simulink model "wtm2"  (R2020a)
settings: Solver=VariableStepAuto  StartTime=0.0  StopTime=10.0  RelTol=1e-3
(part 1 of 8)
settings Model: Creator=kishan  LastModifiedBy=kishan

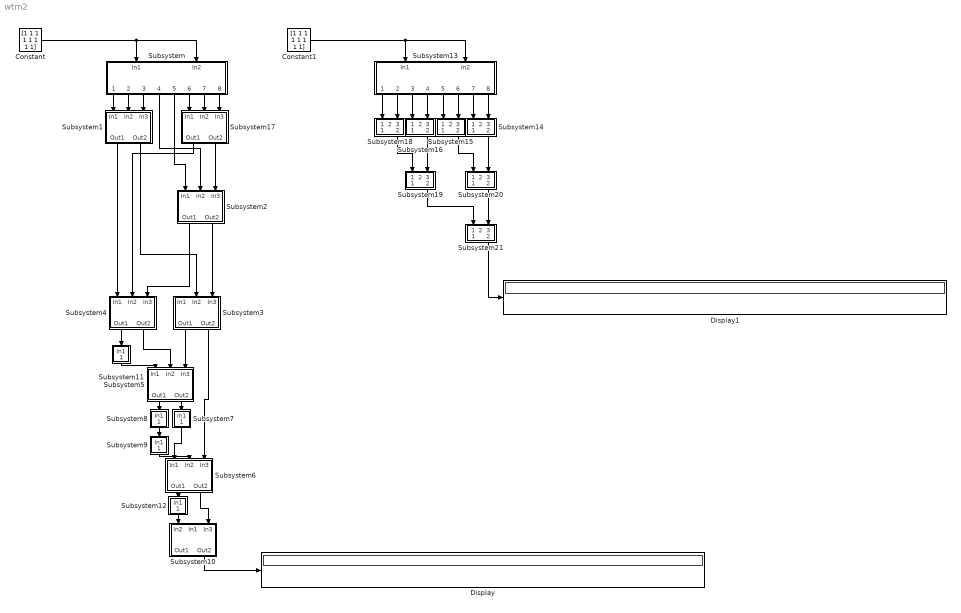
== system wtm2 ==
  Constant : Constant  Value=[1 1 1 1 1 1 1 1]  OutDataTypeStr=boolean
  Constant1 : Constant  Value=[1 1 1 1 1 1 1 1]  OutDataTypeStr=boolean
  Display : Display
  Display1 : Display
  Subsystem : Subsystem
  Subsystem1 : Subsystem
  Subsystem10 : Subsystem
  Subsystem11 : Subsystem
  Subsystem12 : Subsystem
  Subsystem13 : Subsystem
  Subsystem14 : Subsystem
  Subsystem15 : Subsystem
  Subsystem16 : Subsystem
  Subsystem17 : Subsystem
  Subsystem18 : Subsystem
  Subsystem19 : Subsystem
  Subsystem2 : Subsystem
  Subsystem20 : Subsystem
  Subsystem21 : Subsystem
  Subsystem3 : Subsystem
  Subsystem4 : Subsystem
  Subsystem5 : Subsystem
  Subsystem6 : Subsystem
  Subsystem7 : Subsystem
  Subsystem8 : Subsystem
  Subsystem9 : Subsystem
  wires:
  Subsystem/6(Out6) -> Subsystem17/1(In1)
  Subsystem/7(Out7) -> Subsystem17/2(In2)
  Subsystem/8(Out8) -> Subsystem17/3(In3)
  Constant/1 -> Subsystem/2(In2), Subsystem/1(In1)
  Subsystem10/2(Out2) -> Display/1
  Constant1/1 -> Subsystem13/2(In2), Subsystem13/1(In1)
  Subsystem13/8(Out8) -> Subsystem14/3(In3)
  Subsystem13/7(Out7) -> Subsystem14/1(In2)
  Subsystem13/6(Out6) -> Subsystem15/3(In3)
  Subsystem13/5(Out5) -> Subsystem15/1(In2)
  Subsystem13/4(Out4) -> Subsystem16/3(In3)
  Subsystem13/3(Out3) -> Subsystem16/1(In2)
  Subsystem13/2(Out2) -> Subsystem18/3(In3)
  Subsystem13/1(Out1) -> Subsystem18/1(In2)
  Subsystem16/2(Out2) -> Subsystem19/3(In3)
  Subsystem18/2(Out2) -> Subsystem19/1(In2)
  Subsystem14/2(Out2) -> Subsystem20/3(In3)
  Subsystem15/2(Out2) -> Subsystem20/1(In2)
  Subsystem20/2(Out2) -> Subsystem21/3(In3)
  Subsystem19/2(Out2) -> Subsystem21/1(In2)
  Subsystem21/2(Out2) -> Display1/1
  Subsystem/1(Out1) -> Subsystem1/1(In1)
  Subsystem/2(Out2) -> Subsystem1/2(In2)
  Subsystem/3(Out3) -> Subsystem1/3(In3)
  Subsystem17/2(Out2) -> Subsystem2/3(In3)
  Subsystem/5(Out5) -> Subsystem2/1(In1)
  Subsystem2/2(Out2) -> Subsystem3/3(In3)
  Subsystem1/1(Out1) -> Subsystem4/1(In1)
  Subsystem17/1(Out1) -> Subsystem4/2(In2)
  Subsystem2/1(Out1) -> Subsystem4/3(In3)
  Subsystem3/1(Out1) -> Subsystem5/3(In3)
  Subsystem4/2(Out2) -> Subsystem5/2(In2)
  Subsystem4/1(Out1) -> Subsystem11/1(In1)
  Subsystem11/1(Out2) -> Subsystem5/1(In1)
  Subsystem3/2(Out2) -> Subsystem6/3(In3)
  Subsystem5/2(Out2) -> Subsystem7/1(In1)
  Subsystem7/1(Out2) -> Subsystem6/1(In1)
  Subsystem5/1(Out1) -> Subsystem8/1(In1)
  Subsystem8/1(Out2) -> Subsystem9/1(In1)
  Subsystem9/1(Out2) -> Subsystem6/2(In2)
  Subsystem6/2(Out2) -> Subsystem10/3(In3)
  Subsystem6/1(Out1) -> Subsystem12/1(In1)
  Subsystem12/1(Out2) -> Subsystem10/1(In2)
  Subsystem/4(Out4) -> Subsystem2/2(In2)
  Subsystem1/2(Out2) -> Subsystem3/2(In2)

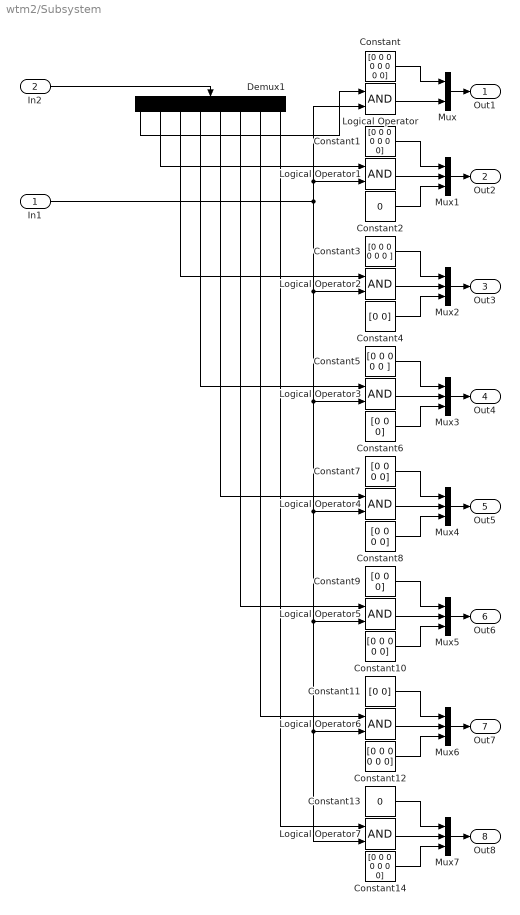
== system wtm2/Subsystem ==
  In1 : Inport
  In2 : Inport  Port=2
  Constant : Constant  Value=[0 0 0 0 0 0 0 0]  OutDataTypeStr=boolean
  Constant1 : Constant  Value=[0 0 0 0 0 0 0]  OutDataTypeStr=boolean
  Constant10 : Constant  Value=[0 0 0 0 0]  OutDataTypeStr=boolean
  Constant11 : Constant  Value=[0 0]  OutDataTypeStr=boolean
  Constant12 : Constant  Value=[0 0 0 0 0 0]  OutDataTypeStr=boolean
  Constant13 : Constant  Value=0  OutDataTypeStr=boolean
  Constant14 : Constant  Value=[0 0 0 0 0 0 0]  OutDataTypeStr=boolean
  Constant2 : Constant  Value=0  OutDataTypeStr=boolean
  Constant3 : Constant  Value=[0 0 0 0 0 0 ]  OutDataTypeStr=boolean
  Constant4 : Constant  Value=[0 0]  OutDataTypeStr=boolean
  Constant5 : Constant  Value=[0 0 0 0 0 ]  OutDataTypeStr=boolean
  Constant6 : Constant  Value=[0 0 0]  OutDataTypeStr=boolean
  Constant7 : Constant  Value=[0 0 0 0]  OutDataTypeStr=boolean
  Constant8 : Constant  Value=[0 0 0 0]  OutDataTypeStr=boolean
  Constant9 : Constant  Value=[0 0 0]  OutDataTypeStr=boolean
  Demux1 : Demux  Outputs=8
  Logical Operator{,1..7} (8 alike) : Logic  AllPortsSameDT=off  OutDataTypeStr=boolean
  Mux : Mux  Inputs=2
  Mux{1..7} (7 alike) : Mux  Inputs=3
  Out1 : Outport
  Out2 : Outport  Port=2
  Out3 : Outport  Port=3
  Out4 : Outport  Port=4
  Out5 : Outport  Port=5
  Out6 : Outport  Port=6
  Out7 : Outport  Port=7
  Out8 : Outport  Port=8
  wires:
  In2/1 -> Demux1/1
  In1/1 -> Logical Operator/2, Logical Operator1/2, Logical Operator2/2, Logical Operator3/2, Logical Operator4/2, Logical Operator5/2, Logical Operator7/2, Logical Operator6/2
  Constant7/1 -> Mux4/1
  Mux3/1 -> Out4/1
  Mux5/1 -> Out6/1
  Constant11/1 -> Mux6/1
  Constant2/1 -> Mux1/3
  Logical Operator3/1 -> Mux3/2
  Mux2/1 -> Out3/1
  Logical Operator2/1 -> Mux2/2
  Constant10/1 -> Mux5/3
  Constant/1 -> Mux/1
  Constant9/1 -> Mux5/1
  Constant4/1 -> Mux2/3
  Constant12/1 -> Mux6/3
  Logical Operator7/1 -> Mux7/2
  Constant8/1 -> Mux4/3
  Constant13/1 -> Mux7/1
  Constant14/1 -> Mux7/3
  Mux1/1 -> Out2/1
  Constant5/1 -> Mux3/1
  Mux6/1 -> Out7/1
  Constant1/1 -> Mux1/1
  Constant3/1 -> Mux2/1
  Mux/1 -> Out1/1
  Logical Operator6/1 -> Mux6/2
  Logical Operator/1 -> Mux/2
  Logical Operator4/1 -> Mux4/2
  Mux7/1 -> Out8/1
  Logical Operator1/1 -> Mux1/2
  Logical Operator5/1 -> Mux5/2
  Mux4/1 -> Out5/1
  Constant6/1 -> Mux3/3
  Demux1/8 -> Logical Operator7/1
  Demux1/7 -> Logical Operator6/1
  Demux1/6 -> Logical Operator5/1
  Demux1/5 -> Logical Operator4/1
  Demux1/4 -> Logical Operator3/1
  Demux1/3 -> Logical Operator2/1
  Demux1/2 -> Logical Operator1/1
  Demux1/1 -> Logical Operator/1

== system wtm2/Subsystem1 ==
  In1 : Inport
  In2 : Inport  Port=2
  In3 : Inport  Port=3
  Demux : Demux  Outputs=16
  Demux1 : Demux  Outputs=16
  Demux2 : Demux  Outputs=16
  Mux : Mux  Inputs=16
  Mux1 : Mux  Inputs=16
  Subsystem1 : Subsystem
  Subsystem10 : Subsystem
  Subsystem11 : Subsystem
  Subsystem12 : Subsystem
  Subsystem13 : Subsystem
  Subsystem14 : Subsystem
  Subsystem15 : Subsystem
  Subsystem16 : Subsystem
  Subsystem2 : Subsystem
  Subsystem3 : Subsystem
  Subsystem4 : Subsystem
  Subsystem5 : Subsystem
  Subsystem6 : Subsystem
  Subsystem7 : Subsystem
  Subsystem8 : Subsystem
  Subsystem9 : Subsystem
  Out1 : Outport
  Out2 : Outport  Port=2
  wires:
  Demux2/2 -> Subsystem2/3(In3)
  Demux/9 -> Subsystem9/1(In1)
  Subsystem7/1(Out1) -> Mux1/7
  Subsystem11/2(Out2) -> Mux/11
  Demux2/8 -> Subsystem8/3(In3)
  Subsystem2/2(Out2) -> Mux/2
  Subsystem1/2(Out2) -> Mux/1
  Demux/7 -> Subsystem7/1(In1)
  Demux2/11 -> Subsystem11/3(In3)
  Demux2/1 -> Subsystem1/3(In3)
  Demux1/10 -> Subsystem10/2(In2)
  Demux2/13 -> Subsystem13/3(In3)
  Subsystem4/2(Out2) -> Mux/4
  Demux1/16 -> Subsystem16/2(In2)
  Demux2/15 -> Subsystem15/3(In3)
  Demux2/3 -> Subsystem3/3(In3)
  Demux2/6 -> Subsystem6/3(In3)
  Mux1/1 -> Out2/1
  Demux/13 -> Subsystem13/1(In1)
  Subsystem14/1(Out1) -> Mux1/14
  Demux1/13 -> Subsystem13/2(In2)
  Subsystem12/1(Out1) -> Mux1/12
  Subsystem1/1(Out1) -> Mux1/1
  Demux1/2 -> Subsystem2/2(In2)
  Subsystem12/2(Out2) -> Mux/12
  Subsystem5/1(Out1) -> Mux1/5
  Demux2/12 -> Subsystem12/3(In3)
  Demux1/14 -> Subsystem14/2(In2)
  Subsystem13/1(Out1) -> Mux1/13
  Demux1/11 -> Subsystem11/2(In2)
  Subsystem7/2(Out2) -> Mux/7
  Demux2/5 -> Subsystem5/3(In3)
  Subsystem10/2(Out2) -> Mux/10
  Demux1/1 -> Subsystem1/2(In2)
  Demux2/10 -> Subsystem10/3(In3)
  Demux1/7 -> Subsystem7/2(In2)
  Subsystem16/1(Out1) -> Mux1/16
  Demux/3 -> Subsystem3/1(In1)
  Demux/14 -> Subsystem14/1(In1)
  Subsystem13/2(Out2) -> Mux/13
  Demux/6 -> Subsystem6/1(In1)
  Demux/11 -> Subsystem11/1(In1)
  Mux/1 -> Out1/1
  Subsystem3/2(Out2) -> Mux/3
  Subsystem2/1(Out1) -> Mux1/2
  Subsystem16/2(Out2) -> Mux/16
  Subsystem9/2(Out2) -> Mux/9
  Subsystem10/1(Out1) -> Mux1/10
  Subsystem6/2(Out2) -> Mux/6
  Demux/2 -> Subsystem2/1(In1)
  Demux1/12 -> Subsystem12/2(In2)
  Demux1/15 -> Subsystem15/2(In2)
  Demux2/14 -> Subsystem14/3(In3)
  Demux1/9 -> Subsystem9/2(In2)
  Subsystem4/1(Out1) -> Mux1/4
  Demux1/8 -> Subsystem8/2(In2)
  Demux/12 -> Subsystem12/1(In1)
  Subsystem3/1(Out1) -> Mux1/3
  In1/1 -> Demux2/1
  In2/1 -> Demux1/1
  Demux/8 -> Subsystem8/1(In1)
  Demux2/16 -> Subsystem16/3(In3)
  Demux1/6 -> Subsystem6/2(In2)
  Subsystem14/2(Out2) -> Mux/14
  Demux1/4 -> Subsystem4/2(In2)
  Demux/16 -> Subsystem16/1(In1)
  Subsystem9/1(Out1) -> Mux1/9
  Demux/4 -> Subsystem4/1(In1)
  Demux/15 -> Subsystem15/1(In1)
  Subsystem5/2(Out2) -> Mux/5
  Demux/1 -> Subsystem1/1(In1)
  Demux1/5 -> Subsystem5/2(In2)
  Subsystem15/1(Out1) -> Mux1/15
  Demux/10 -> Subsystem10/1(In1)
  Subsystem15/2(Out2) -> Mux/15
  Demux2/9 -> Subsystem9/3(In3)
  Subsystem6/1(Out1) -> Mux1/6
  Subsystem8/2(Out2) -> Mux/8
  Subsystem8/1(Out1) -> Mux1/8
  Demux2/7 -> Subsystem7/3(In3)
  In3/1 -> Demux/1
  Subsystem11/1(Out1) -> Mux1/11
  Demux1/3 -> Subsystem3/2(In2)
  Demux2/4 -> Subsystem4/3(In3)
  Demux/5 -> Subsystem5/1(In1)

== system wtm2/Subsystem10 ==
  In2 : Inport
  In1 : Inport  Port=2
  In3 : Inport  Port=3
  Demux : Demux  Outputs=16
  Demux1 : Demux  Outputs=16
  Mux : Mux  Inputs=16
  Subsystem4 : Subsystem
  Subsystem5 : Subsystem
  Subsystem6 : Subsystem
  Subsystem7 : Subsystem
  Out1 : Outport
  Out2 : Outport  Port=2
  wires:
  Demux/11 -> Subsystem5/3(In3)
  Subsystem4/4(Out4) -> Mux/15
  Demux1/4 -> Subsystem7/9(In9)
  Demux/14 -> Subsystem4/2(In2)
  Subsystem7/4(Out4) -> Mux/3
  Subsystem7/1(Out1) -> Out1/1
  Subsystem7/3(Out3) -> Mux/2
  Demux/3 -> Subsystem7/3(In3)
  Demux/15 -> Subsystem4/3(In3)
  Subsystem6/1(Out1) -> Subsystem7/5(In5)
  In3/1 -> Demux1/1
  Subsystem4/5(Out5) -> Mux/16
  Subsystem4/3(Out3) -> Mux/14
  Demux1/15 -> Subsystem4/8(In8)
  Subsystem5/4(Out4) -> Mux/11
  Subsystem5/1(Out1) -> Subsystem6/5(In5)
  Subsystem5/3(Out3) -> Mux/10
  Demux1/16 -> Subsystem4/9(In9)
  Demux/9 -> Subsystem5/1(In1)
  Subsystem7/5(Out5) -> Mux/4
  Demux1/3 -> Subsystem7/8(In8)
  Demux1/9 -> Subsystem5/6(In6)
  Subsystem6/5(Out5) -> Mux/8
  Demux/1 -> Subsystem7/1(In1)
  Demux1/13 -> Subsystem4/6(In6)
  Demux/5 -> Subsystem6/1(In1)
  Demux1/7 -> Subsystem6/8(In8)
  In2/1 -> Demux/1
  Demux1/12 -> Subsystem5/9(In9)
  Subsystem6/4(Out4) -> Mux/7
  Subsystem5/5(Out5) -> Mux/12
  Mux/1 -> Out2/1
  Subsystem6/3(Out3) -> Mux/6
  Demux1/8 -> Subsystem6/9(In9)
  Demux/12 -> Subsystem5/4(In4)
  Subsystem4/1(Out1) -> Subsystem5/5(In5)
  Demux/6 -> Subsystem6/2(In2)
  Subsystem6/2(Out2) -> Mux/5
  Demux1/1 -> Subsystem7/6(In6)
  Demux/8 -> Subsystem6/4(In4)
  Demux1/5 -> Subsystem6/6(In6)
  Demux/7 -> Subsystem6/3(In3)
  Demux/4 -> Subsystem7/4(In4)
  Demux/10 -> Subsystem5/2(In2)
  Subsystem5/2(Out2) -> Mux/9
  Demux/2 -> Subsystem7/2(In2)
  Demux1/6 -> Subsystem6/7(In7)
  Subsystem7/2(Out2) -> Mux/1
  Subsystem4/2(Out2) -> Mux/13
  Demux/13 -> Subsystem4/1(In1)
  Demux1/11 -> Subsystem5/8(In8)
  Demux1/2 -> Subsystem7/7(In7)
  Demux1/14 -> Subsystem4/7(In7)
  Demux/16 -> Subsystem4/4(In4)
  Demux1/10 -> Subsystem5/7(In7)
  In1/1 -> Subsystem4/5(In5)

== system wtm2/Subsystem11 ==
  In1 : Inport
  Constant : Constant  Value=0  OutDataTypeStr=boolean
  Demux : Demux  Outputs=16
  Display : Display
  Mux : Mux  Inputs=16
  Out2 : Outport
  wires:
  Demux/5 -> Mux/6
  Demux/6 -> Mux/7
  Demux/4 -> Mux/5
  Demux/10 -> Mux/11
  In1/1 -> Demux/1
  Constant/1 -> Mux/1
  Demux/15 -> Mux/16
  Mux/1 -> Out2/1
  Demux/1 -> Mux/2
  Demux/9 -> Mux/10
  Demux/2 -> Mux/3
  Demux/11 -> Mux/12
  Demux/12 -> Mux/13
  Demux/14 -> Mux/15
  Demux/13 -> Mux/14
  Demux/3 -> Mux/4
  Demux/8 -> Mux/9
  Demux/7 -> Mux/8
  Demux/16 -> Display/1

== system wtm2/Subsystem12 ==
  In1 : Inport
  Constant : Constant  Value=0  OutDataTypeStr=boolean
  Demux : Demux  Outputs=16
  Display : Display
  Mux : Mux  Inputs=16
  Out2 : Outport
  wires:
  Demux/5 -> Mux/6
  Demux/6 -> Mux/7
  Demux/4 -> Mux/5
  Demux/10 -> Mux/11
  In1/1 -> Demux/1
  Constant/1 -> Mux/1
  Demux/15 -> Mux/16
  Mux/1 -> Out2/1
  Demux/1 -> Mux/2
  Demux/9 -> Mux/10
  Demux/2 -> Mux/3
  Demux/11 -> Mux/12
  Demux/12 -> Mux/13
  Demux/14 -> Mux/15
  Demux/13 -> Mux/14
  Demux/3 -> Mux/4
  Demux/8 -> Mux/9
  Demux/7 -> Mux/8
  Demux/16 -> Display/1

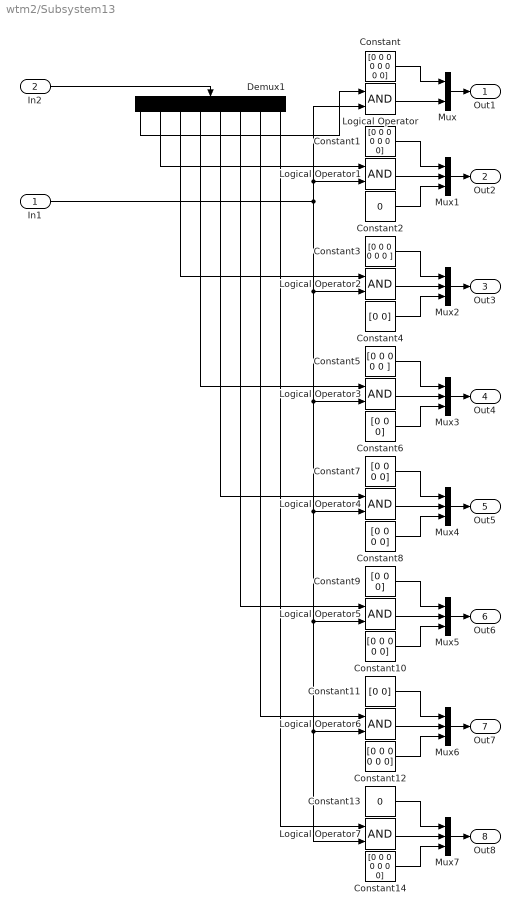
== system wtm2/Subsystem13 ==
  In1 : Inport
  In2 : Inport  Port=2
  Constant : Constant  Value=[0 0 0 0 0 0 0 0]  OutDataTypeStr=boolean
  Constant1 : Constant  Value=[0 0 0 0 0 0 0]  OutDataTypeStr=boolean
  Constant10 : Constant  Value=[0 0 0 0 0]  OutDataTypeStr=boolean
  Constant11 : Constant  Value=[0 0]  OutDataTypeStr=boolean
  Constant12 : Constant  Value=[0 0 0 0 0 0]  OutDataTypeStr=boolean
  Constant13 : Constant  Value=0  OutDataTypeStr=boolean
  Constant14 : Constant  Value=[0 0 0 0 0 0 0]  OutDataTypeStr=boolean
  Constant2 : Constant  Value=0  OutDataTypeStr=boolean
  Constant3 : Constant  Value=[0 0 0 0 0 0 ]  OutDataTypeStr=boolean
  Constant4 : Constant  Value=[0 0]  OutDataTypeStr=boolean
  Constant5 : Constant  Value=[0 0 0 0 0 ]  OutDataTypeStr=boolean
  Constant6 : Constant  Value=[0 0 0]  OutDataTypeStr=boolean
  Constant7 : Constant  Value=[0 0 0 0]  OutDataTypeStr=boolean
  Constant8 : Constant  Value=[0 0 0 0]  OutDataTypeStr=boolean
  Constant9 : Constant  Value=[0 0 0]  OutDataTypeStr=boolean
  Demux1 : Demux  Outputs=8
  Logical Operator{,1..7} (8 alike) : Logic  AllPortsSameDT=off  OutDataTypeStr=boolean
  Mux : Mux  Inputs=2
  Mux{1..7} (7 alike) : Mux  Inputs=3
  Out1 : Outport
  Out2 : Outport  Port=2
  Out3 : Outport  Port=3
  Out4 : Outport  Port=4
  Out5 : Outport  Port=5
  Out6 : Outport  Port=6
  Out7 : Outport  Port=7
  Out8 : Outport  Port=8
  wires:
  In2/1 -> Demux1/1
  In1/1 -> Logical Operator/2, Logical Operator1/2, Logical Operator2/2, Logical Operator3/2, Logical Operator4/2, Logical Operator5/2, Logical Operator7/2, Logical Operator6/2
  Constant7/1 -> Mux4/1
  Mux3/1 -> Out4/1
  Mux5/1 -> Out6/1
  Constant11/1 -> Mux6/1
  Constant2/1 -> Mux1/3
  Logical Operator3/1 -> Mux3/2
  Mux2/1 -> Out3/1
  Logical Operator2/1 -> Mux2/2
  Constant10/1 -> Mux5/3
  Constant/1 -> Mux/1
  Constant9/1 -> Mux5/1
  Constant4/1 -> Mux2/3
  Constant12/1 -> Mux6/3
  Logical Operator7/1 -> Mux7/2
  Constant8/1 -> Mux4/3
  Constant13/1 -> Mux7/1
  Constant14/1 -> Mux7/3
  Mux1/1 -> Out2/1
  Constant5/1 -> Mux3/1
  Mux6/1 -> Out7/1
  Constant1/1 -> Mux1/1
  Constant3/1 -> Mux2/1
  Mux/1 -> Out1/1
  Logical Operator6/1 -> Mux6/2
  Logical Operator/1 -> Mux/2
  Logical Operator4/1 -> Mux4/2
  Mux7/1 -> Out8/1
  Logical Operator1/1 -> Mux1/2
  Logical Operator5/1 -> Mux5/2
  Mux4/1 -> Out5/1
  Constant6/1 -> Mux3/3
  Demux1/8 -> Logical Operator7/1
  Demux1/7 -> Logical Operator6/1
  Demux1/6 -> Logical Operator5/1
  Demux1/5 -> Logical Operator4/1
  Demux1/4 -> Logical Operator3/1
  Demux1/3 -> Logical Operator2/1
  Demux1/2 -> Logical Operator1/1
  Demux1/1 -> Logical Operator/1

== system wtm2/Subsystem14 ==
  In2 : Inport
  In1 : Inport  Port=2
  In3 : Inport  Port=3
  Demux : Demux  Outputs=16
  Demux1 : Demux  Outputs=16
  Mux : Mux  Inputs=16
  Subsystem4 : Subsystem
  Subsystem5 : Subsystem
  Subsystem6 : Subsystem
  Subsystem7 : Subsystem
  Out1 : Outport
  Out2 : Outport  Port=2
  wires:
  Demux/11 -> Subsystem5/3(In3)
  Subsystem4/4(Out4) -> Mux/15
  Demux1/4 -> Subsystem7/9(In9)
  Demux/14 -> Subsystem4/2(In2)
  Subsystem7/4(Out4) -> Mux/3
  Subsystem7/1(Out1) -> Out1/1
  Subsystem7/3(Out3) -> Mux/2
  Demux/3 -> Subsystem7/3(In3)
  Demux/15 -> Subsystem4/3(In3)
  Subsystem6/1(Out1) -> Subsystem7/5(In5)
  In3/1 -> Demux1/1
  Subsystem4/5(Out5) -> Mux/16
  Subsystem4/3(Out3) -> Mux/14
  Demux1/15 -> Subsystem4/8(In8)
  Subsystem5/4(Out4) -> Mux/11
  Subsystem5/1(Out1) -> Subsystem6/5(In5)
  Subsystem5/3(Out3) -> Mux/10
  Demux1/16 -> Subsystem4/9(In9)
  Demux/9 -> Subsystem5/1(In1)
  Subsystem7/5(Out5) -> Mux/4
  Demux1/3 -> Subsystem7/8(In8)
  Demux1/9 -> Subsystem5/6(In6)
  Subsystem6/5(Out5) -> Mux/8
  Demux/1 -> Subsystem7/1(In1)
  Demux1/13 -> Subsystem4/6(In6)
  Demux/5 -> Subsystem6/1(In1)
  Demux1/7 -> Subsystem6/8(In8)
  In2/1 -> Demux/1
  Demux1/12 -> Subsystem5/9(In9)
  Subsystem6/4(Out4) -> Mux/7
  Subsystem5/5(Out5) -> Mux/12
  Mux/1 -> Out2/1
  Subsystem6/3(Out3) -> Mux/6
  Demux1/8 -> Subsystem6/9(In9)
  Demux/12 -> Subsystem5/4(In4)
  Subsystem4/1(Out1) -> Subsystem5/5(In5)
  Demux/6 -> Subsystem6/2(In2)
  Subsystem6/2(Out2) -> Mux/5
  Demux1/1 -> Subsystem7/6(In6)
  Demux/8 -> Subsystem6/4(In4)
  Demux1/5 -> Subsystem6/6(In6)
  Demux/7 -> Subsystem6/3(In3)
  Demux/4 -> Subsystem7/4(In4)
  Demux/10 -> Subsystem5/2(In2)
  Subsystem5/2(Out2) -> Mux/9
  Demux/2 -> Subsystem7/2(In2)
  Demux1/6 -> Subsystem6/7(In7)
  Subsystem7/2(Out2) -> Mux/1
  Subsystem4/2(Out2) -> Mux/13
  Demux/13 -> Subsystem4/1(In1)
  Demux1/11 -> Subsystem5/8(In8)
  Demux1/2 -> Subsystem7/7(In7)
  Demux1/14 -> Subsystem4/7(In7)
  Demux/16 -> Subsystem4/4(In4)
  Demux1/10 -> Subsystem5/7(In7)
  In1/1 -> Subsystem4/5(In5)

== system wtm2/Subsystem15 ==
  In2 : Inport
  In1 : Inport  Port=2
  In3 : Inport  Port=3
  Demux : Demux  Outputs=16
  Demux1 : Demux  Outputs=16
  Mux : Mux  Inputs=16
  Subsystem4 : Subsystem
  Subsystem5 : Subsystem
  Subsystem6 : Subsystem
  Subsystem7 : Subsystem
  Out1 : Outport
  Out2 : Outport  Port=2
  wires:
  Demux/11 -> Subsystem5/3(In3)
  Subsystem4/4(Out4) -> Mux/15
  Demux1/4 -> Subsystem7/9(In9)
  Demux/14 -> Subsystem4/2(In2)
  Subsystem7/4(Out4) -> Mux/3
  Subsystem7/1(Out1) -> Out1/1
  Subsystem7/3(Out3) -> Mux/2
  Demux/3 -> Subsystem7/3(In3)
  Demux/15 -> Subsystem4/3(In3)
  Subsystem6/1(Out1) -> Subsystem7/5(In5)
  In3/1 -> Demux1/1
  Subsystem4/5(Out5) -> Mux/16
  Subsystem4/3(Out3) -> Mux/14
  Demux1/15 -> Subsystem4/8(In8)
  Subsystem5/4(Out4) -> Mux/11
  Subsystem5/1(Out1) -> Subsystem6/5(In5)
  Subsystem5/3(Out3) -> Mux/10
  Demux1/16 -> Subsystem4/9(In9)
  Demux/9 -> Subsystem5/1(In1)
  Subsystem7/5(Out5) -> Mux/4
  Demux1/3 -> Subsystem7/8(In8)
  Demux1/9 -> Subsystem5/6(In6)
  Subsystem6/5(Out5) -> Mux/8
  Demux/1 -> Subsystem7/1(In1)
  Demux1/13 -> Subsystem4/6(In6)
  Demux/5 -> Subsystem6/1(In1)
  Demux1/7 -> Subsystem6/8(In8)
  In2/1 -> Demux/1
  Demux1/12 -> Subsystem5/9(In9)
  Subsystem6/4(Out4) -> Mux/7
  Subsystem5/5(Out5) -> Mux/12
  Mux/1 -> Out2/1
  Subsystem6/3(Out3) -> Mux/6
  Demux1/8 -> Subsystem6/9(In9)
  Demux/12 -> Subsystem5/4(In4)
  Subsystem4/1(Out1) -> Subsystem5/5(In5)
  Demux/6 -> Subsystem6/2(In2)
  Subsystem6/2(Out2) -> Mux/5
  Demux1/1 -> Subsystem7/6(In6)
  Demux/8 -> Subsystem6/4(In4)
  Demux1/5 -> Subsystem6/6(In6)
  Demux/7 -> Subsystem6/3(In3)
  Demux/4 -> Subsystem7/4(In4)
  Demux/10 -> Subsystem5/2(In2)
  Subsystem5/2(Out2) -> Mux/9
  Demux/2 -> Subsystem7/2(In2)
  Demux1/6 -> Subsystem6/7(In7)
  Subsystem7/2(Out2) -> Mux/1
  Subsystem4/2(Out2) -> Mux/13
  Demux/13 -> Subsystem4/1(In1)
  Demux1/11 -> Subsystem5/8(In8)
  Demux1/2 -> Subsystem7/7(In7)
  Demux1/14 -> Subsystem4/7(In7)
  Demux/16 -> Subsystem4/4(In4)
  Demux1/10 -> Subsystem5/7(In7)
  In1/1 -> Subsystem4/5(In5)

== system wtm2/Subsystem16 ==
  In2 : Inport
  In1 : Inport  Port=2
  In3 : Inport  Port=3
  Demux : Demux  Outputs=16
  Demux1 : Demux  Outputs=16
  Mux : Mux  Inputs=16
  Subsystem4 : Subsystem
  Subsystem5 : Subsystem
  Subsystem6 : Subsystem
  Subsystem7 : Subsystem
  Out1 : Outport
  Out2 : Outport  Port=2
  wires:
  Demux/11 -> Subsystem5/3(In3)
  Subsystem4/4(Out4) -> Mux/15
  Demux1/4 -> Subsystem7/9(In9)
  Demux/14 -> Subsystem4/2(In2)
  Subsystem7/4(Out4) -> Mux/3
  Subsystem7/1(Out1) -> Out1/1
  Subsystem7/3(Out3) -> Mux/2
  Demux/3 -> Subsystem7/3(In3)
  Demux/15 -> Subsystem4/3(In3)
  Subsystem6/1(Out1) -> Subsystem7/5(In5)
  In3/1 -> Demux1/1
  Subsystem4/5(Out5) -> Mux/16
  Subsystem4/3(Out3) -> Mux/14
  Demux1/15 -> Subsystem4/8(In8)
  Subsystem5/4(Out4) -> Mux/11
  Subsystem5/1(Out1) -> Subsystem6/5(In5)
  Subsystem5/3(Out3) -> Mux/10
  Demux1/16 -> Subsystem4/9(In9)
  Demux/9 -> Subsystem5/1(In1)
  Subsystem7/5(Out5) -> Mux/4
  Demux1/3 -> Subsystem7/8(In8)
  Demux1/9 -> Subsystem5/6(In6)
  Subsystem6/5(Out5) -> Mux/8
  Demux/1 -> Subsystem7/1(In1)
  Demux1/13 -> Subsystem4/6(In6)
  Demux/5 -> Subsystem6/1(In1)
  Demux1/7 -> Subsystem6/8(In8)
  In2/1 -> Demux/1
  Demux1/12 -> Subsystem5/9(In9)
  Subsystem6/4(Out4) -> Mux/7
  Subsystem5/5(Out5) -> Mux/12
  Mux/1 -> Out2/1
  Subsystem6/3(Out3) -> Mux/6
  Demux1/8 -> Subsystem6/9(In9)
  Demux/12 -> Subsystem5/4(In4)
  Subsystem4/1(Out1) -> Subsystem5/5(In5)
  Demux/6 -> Subsystem6/2(In2)
  Subsystem6/2(Out2) -> Mux/5
  Demux1/1 -> Subsystem7/6(In6)
  Demux/8 -> Subsystem6/4(In4)
  Demux1/5 -> Subsystem6/6(In6)
  Demux/7 -> Subsystem6/3(In3)
  Demux/4 -> Subsystem7/4(In4)
  Demux/10 -> Subsystem5/2(In2)
  Subsystem5/2(Out2) -> Mux/9
  Demux/2 -> Subsystem7/2(In2)
  Demux1/6 -> Subsystem6/7(In7)
  Subsystem7/2(Out2) -> Mux/1
  Subsystem4/2(Out2) -> Mux/13
  Demux/13 -> Subsystem4/1(In1)
  Demux1/11 -> Subsystem5/8(In8)
  Demux1/2 -> Subsystem7/7(In7)
  Demux1/14 -> Subsystem4/7(In7)
  Demux/16 -> Subsystem4/4(In4)
  Demux1/10 -> Subsystem5/7(In7)
  In1/1 -> Subsystem4/5(In5)

== system wtm2/Subsystem17 ==
  In1 : Inport
  In2 : Inport  Port=2
  In3 : Inport  Port=3
  Demux : Demux  Outputs=16
  Demux1 : Demux  Outputs=16
  Demux2 : Demux  Outputs=16
  Mux : Mux  Inputs=16
  Mux1 : Mux  Inputs=16
  Subsystem1 : Subsystem
  Subsystem10 : Subsystem
  Subsystem11 : Subsystem
  Subsystem12 : Subsystem
  Subsystem13 : Subsystem
  Subsystem14 : Subsystem
  Subsystem15 : Subsystem
  Subsystem16 : Subsystem
  Subsystem2 : Subsystem
  Subsystem3 : Subsystem
  Subsystem4 : Subsystem
  Subsystem5 : Subsystem
  Subsystem6 : Subsystem
  Subsystem7 : Subsystem
  Subsystem8 : Subsystem
  Subsystem9 : Subsystem
  Out1 : Outport
  Out2 : Outport  Port=2
  wires:
  Demux2/2 -> Subsystem2/3(In3)
  Demux/9 -> Subsystem9/1(In1)
  Subsystem7/1(Out1) -> Mux1/7
  Subsystem11/2(Out2) -> Mux/11
  Demux2/8 -> Subsystem8/3(In3)
  Subsystem2/2(Out2) -> Mux/2
  Subsystem1/2(Out2) -> Mux/1
  Demux/7 -> Subsystem7/1(In1)
  Demux2/11 -> Subsystem11/3(In3)
  Demux2/1 -> Subsystem1/3(In3)
  Demux1/10 -> Subsystem10/2(In2)
  Demux2/13 -> Subsystem13/3(In3)
  Subsystem4/2(Out2) -> Mux/4
  Demux1/16 -> Subsystem16/2(In2)
  Demux2/15 -> Subsystem15/3(In3)
  Demux2/3 -> Subsystem3/3(In3)
  Demux2/6 -> Subsystem6/3(In3)
  Mux1/1 -> Out2/1
  Demux/13 -> Subsystem13/1(In1)
  Subsystem14/1(Out1) -> Mux1/14
  Demux1/13 -> Subsystem13/2(In2)
  Subsystem12/1(Out1) -> Mux1/12
  Subsystem1/1(Out1) -> Mux1/1
  Demux1/2 -> Subsystem2/2(In2)
  Subsystem12/2(Out2) -> Mux/12
  Subsystem5/1(Out1) -> Mux1/5
  Demux2/12 -> Subsystem12/3(In3)
  Demux1/14 -> Subsystem14/2(In2)
  Subsystem13/1(Out1) -> Mux1/13
  Demux1/11 -> Subsystem11/2(In2)
  Subsystem7/2(Out2) -> Mux/7
  Demux2/5 -> Subsystem5/3(In3)
  Subsystem10/2(Out2) -> Mux/10
  Demux1/1 -> Subsystem1/2(In2)
  Demux2/10 -> Subsystem10/3(In3)
  Demux1/7 -> Subsystem7/2(In2)
  Subsystem16/1(Out1) -> Mux1/16
  Demux/3 -> Subsystem3/1(In1)
  Demux/14 -> Subsystem14/1(In1)
  Subsystem13/2(Out2) -> Mux/13
  Demux/6 -> Subsystem6/1(In1)
  Demux/11 -> Subsystem11/1(In1)
  Mux/1 -> Out1/1
  Subsystem3/2(Out2) -> Mux/3
  Subsystem2/1(Out1) -> Mux1/2
  Subsystem16/2(Out2) -> Mux/16
  Subsystem9/2(Out2) -> Mux/9
  Subsystem10/1(Out1) -> Mux1/10
  Subsystem6/2(Out2) -> Mux/6
  Demux/2 -> Subsystem2/1(In1)
  Demux1/12 -> Subsystem12/2(In2)
  Demux1/15 -> Subsystem15/2(In2)
  Demux2/14 -> Subsystem14/3(In3)
  Demux1/9 -> Subsystem9/2(In2)
  Subsystem4/1(Out1) -> Mux1/4
  Demux1/8 -> Subsystem8/2(In2)
  Demux/12 -> Subsystem12/1(In1)
  Subsystem3/1(Out1) -> Mux1/3
  In1/1 -> Demux2/1
  In2/1 -> Demux1/1
  Demux/8 -> Subsystem8/1(In1)
  Demux2/16 -> Subsystem16/3(In3)
  Demux1/6 -> Subsystem6/2(In2)
  Subsystem14/2(Out2) -> Mux/14
  Demux1/4 -> Subsystem4/2(In2)
  Demux/16 -> Subsystem16/1(In1)
  Subsystem9/1(Out1) -> Mux1/9
  Demux/4 -> Subsystem4/1(In1)
  Demux/15 -> Subsystem15/1(In1)
  Subsystem5/2(Out2) -> Mux/5
  Demux/1 -> Subsystem1/1(In1)
  Demux1/5 -> Subsystem5/2(In2)
  Subsystem15/1(Out1) -> Mux1/15
  Demux/10 -> Subsystem10/1(In1)
  Subsystem15/2(Out2) -> Mux/15
  Demux2/9 -> Subsystem9/3(In3)
  Subsystem6/1(Out1) -> Mux1/6
  Subsystem8/2(Out2) -> Mux/8
  Subsystem8/1(Out1) -> Mux1/8
  Demux2/7 -> Subsystem7/3(In3)
  In3/1 -> Demux/1
  Subsystem11/1(Out1) -> Mux1/11
  Demux1/3 -> Subsystem3/2(In2)
  Demux2/4 -> Subsystem4/3(In3)
  Demux/5 -> Subsystem5/1(In1)

== system wtm2/Subsystem18 ==
  In2 : Inport
  In1 : Inport  Port=2
  In3 : Inport  Port=3
  Demux : Demux  Outputs=16
  Demux1 : Demux  Outputs=16
  Mux : Mux  Inputs=16
  Subsystem4 : Subsystem
  Subsystem5 : Subsystem
  Subsystem6 : Subsystem
  Subsystem7 : Subsystem
  Out1 : Outport
  Out2 : Outport  Port=2
  wires:
  Demux/11 -> Subsystem5/3(In3)
  Subsystem4/4(Out4) -> Mux/15
  Demux1/4 -> Subsystem7/9(In9)
  Demux/14 -> Subsystem4/2(In2)
  Subsystem7/4(Out4) -> Mux/3
  Subsystem7/1(Out1) -> Out1/1
  Subsystem7/3(Out3) -> Mux/2
  Demux/3 -> Subsystem7/3(In3)
  Demux/15 -> Subsystem4/3(In3)
  Subsystem6/1(Out1) -> Subsystem7/5(In5)
  In3/1 -> Demux1/1
  Subsystem4/5(Out5) -> Mux/16
  Subsystem4/3(Out3) -> Mux/14
  Demux1/15 -> Subsystem4/8(In8)
  Subsystem5/4(Out4) -> Mux/11
  Subsystem5/1(Out1) -> Subsystem6/5(In5)
  Subsystem5/3(Out3) -> Mux/10
  Demux1/16 -> Subsystem4/9(In9)
  Demux/9 -> Subsystem5/1(In1)
  Subsystem7/5(Out5) -> Mux/4
  Demux1/3 -> Subsystem7/8(In8)
  Demux1/9 -> Subsystem5/6(In6)
  Subsystem6/5(Out5) -> Mux/8
  Demux/1 -> Subsystem7/1(In1)
  Demux1/13 -> Subsystem4/6(In6)
  Demux/5 -> Subsystem6/1(In1)
  Demux1/7 -> Subsystem6/8(In8)
  In2/1 -> Demux/1
  Demux1/12 -> Subsystem5/9(In9)
  Subsystem6/4(Out4) -> Mux/7
  Subsystem5/5(Out5) -> Mux/12
  Mux/1 -> Out2/1
  Subsystem6/3(Out3) -> Mux/6
  Demux1/8 -> Subsystem6/9(In9)
  Demux/12 -> Subsystem5/4(In4)
  Subsystem4/1(Out1) -> Subsystem5/5(In5)
  Demux/6 -> Subsystem6/2(In2)
  Subsystem6/2(Out2) -> Mux/5
  Demux1/1 -> Subsystem7/6(In6)
  Demux/8 -> Subsystem6/4(In4)
  Demux1/5 -> Subsystem6/6(In6)
  Demux/7 -> Subsystem6/3(In3)
  Demux/4 -> Subsystem7/4(In4)
  Demux/10 -> Subsystem5/2(In2)
  Subsystem5/2(Out2) -> Mux/9
  Demux/2 -> Subsystem7/2(In2)
  Demux1/6 -> Subsystem6/7(In7)
  Subsystem7/2(Out2) -> Mux/1
  Subsystem4/2(Out2) -> Mux/13
  Demux/13 -> Subsystem4/1(In1)
  Demux1/11 -> Subsystem5/8(In8)
  Demux1/2 -> Subsystem7/7(In7)
  Demux1/14 -> Subsystem4/7(In7)
  Demux/16 -> Subsystem4/4(In4)
  Demux1/10 -> Subsystem5/7(In7)
  In1/1 -> Subsystem4/5(In5)

== system wtm2/Subsystem19 ==
  In2 : Inport
  In1 : Inport  Port=2
  In3 : Inport  Port=3
  Demux : Demux  Outputs=16
  Demux1 : Demux  Outputs=16
  Mux : Mux  Inputs=16
  Subsystem4 : Subsystem
  Subsystem5 : Subsystem
  Subsystem6 : Subsystem
  Subsystem7 : Subsystem
  Out1 : Outport
  Out2 : Outport  Port=2
  wires:
  Demux/11 -> Subsystem5/3(In3)
  Subsystem4/4(Out4) -> Mux/15
  Demux1/4 -> Subsystem7/9(In9)
  Demux/14 -> Subsystem4/2(In2)
  Subsystem7/4(Out4) -> Mux/3
  Subsystem7/1(Out1) -> Out1/1
  Subsystem7/3(Out3) -> Mux/2
  Demux/3 -> Subsystem7/3(In3)
  Demux/15 -> Subsystem4/3(In3)
  Subsystem6/1(Out1) -> Subsystem7/5(In5)
  In3/1 -> Demux1/1
  Subsystem4/5(Out5) -> Mux/16
  Subsystem4/3(Out3) -> Mux/14
  Demux1/15 -> Subsystem4/8(In8)
  Subsystem5/4(Out4) -> Mux/11
  Subsystem5/1(Out1) -> Subsystem6/5(In5)
  Subsystem5/3(Out3) -> Mux/10
  Demux1/16 -> Subsystem4/9(In9)
  Demux/9 -> Subsystem5/1(In1)
  Subsystem7/5(Out5) -> Mux/4
  Demux1/3 -> Subsystem7/8(In8)
  Demux1/9 -> Subsystem5/6(In6)
  Subsystem6/5(Out5) -> Mux/8
  Demux/1 -> Subsystem7/1(In1)
  Demux1/13 -> Subsystem4/6(In6)
  Demux/5 -> Subsystem6/1(In1)
  Demux1/7 -> Subsystem6/8(In8)
  In2/1 -> Demux/1
  Demux1/12 -> Subsystem5/9(In9)
  Subsystem6/4(Out4) -> Mux/7
  Subsystem5/5(Out5) -> Mux/12
  Mux/1 -> Out2/1
  Subsystem6/3(Out3) -> Mux/6
  Demux1/8 -> Subsystem6/9(In9)
  Demux/12 -> Subsystem5/4(In4)
  Subsystem4/1(Out1) -> Subsystem5/5(In5)
  Demux/6 -> Subsystem6/2(In2)
  Subsystem6/2(Out2) -> Mux/5
  Demux1/1 -> Subsystem7/6(In6)
  Demux/8 -> Subsystem6/4(In4)
  Demux1/5 -> Subsystem6/6(In6)
  Demux/7 -> Subsystem6/3(In3)
  Demux/4 -> Subsystem7/4(In4)
  Demux/10 -> Subsystem5/2(In2)
  Subsystem5/2(Out2) -> Mux/9
  Demux/2 -> Subsystem7/2(In2)
  Demux1/6 -> Subsystem6/7(In7)
  Subsystem7/2(Out2) -> Mux/1
  Subsystem4/2(Out2) -> Mux/13
  Demux/13 -> Subsystem4/1(In1)
  Demux1/11 -> Subsystem5/8(In8)
  Demux1/2 -> Subsystem7/7(In7)
  Demux1/14 -> Subsystem4/7(In7)
  Demux/16 -> Subsystem4/4(In4)
  Demux1/10 -> Subsystem5/7(In7)
  In1/1 -> Subsystem4/5(In5)

== system wtm2/Subsystem2 ==
  In1 : Inport
  In2 : Inport  Port=2
  In3 : Inport  Port=3
  Demux : Demux  Outputs=16
  Demux1 : Demux  Outputs=16
  Demux2 : Demux  Outputs=16
  Mux : Mux  Inputs=16
  Mux1 : Mux  Inputs=16
  Subsystem1 : Subsystem
  Subsystem10 : Subsystem
  Subsystem11 : Subsystem
  Subsystem12 : Subsystem
  Subsystem13 : Subsystem
  Subsystem14 : Subsystem
  Subsystem15 : Subsystem
  Subsystem16 : Subsystem
  Subsystem2 : Subsystem
  Subsystem3 : Subsystem
  Subsystem4 : Subsystem
  Subsystem5 : Subsystem
  Subsystem6 : Subsystem
  Subsystem7 : Subsystem
  Subsystem8 : Subsystem
  Subsystem9 : Subsystem
  Out1 : Outport
  Out2 : Outport  Port=2
  wires:
  Demux2/2 -> Subsystem2/3(In3)
  Demux/9 -> Subsystem9/1(In1)
  Subsystem7/1(Out1) -> Mux1/7
  Subsystem11/2(Out2) -> Mux/11
  Demux2/8 -> Subsystem8/3(In3)
  Subsystem2/2(Out2) -> Mux/2
  Subsystem1/2(Out2) -> Mux/1
  Demux/7 -> Subsystem7/1(In1)
  Demux2/11 -> Subsystem11/3(In3)
  Demux2/1 -> Subsystem1/3(In3)
  Demux1/10 -> Subsystem10/2(In2)
  Demux2/13 -> Subsystem13/3(In3)
  Subsystem4/2(Out2) -> Mux/4
  Demux1/16 -> Subsystem16/2(In2)
  Demux2/15 -> Subsystem15/3(In3)
  Demux2/3 -> Subsystem3/3(In3)
  Demux2/6 -> Subsystem6/3(In3)
  Mux1/1 -> Out2/1
  Demux/13 -> Subsystem13/1(In1)
  Subsystem14/1(Out1) -> Mux1/14
  Demux1/13 -> Subsystem13/2(In2)
  Subsystem12/1(Out1) -> Mux1/12
  Subsystem1/1(Out1) -> Mux1/1
  Demux1/2 -> Subsystem2/2(In2)
  Subsystem12/2(Out2) -> Mux/12
  Subsystem5/1(Out1) -> Mux1/5
  Demux2/12 -> Subsystem12/3(In3)
  Demux1/14 -> Subsystem14/2(In2)
  Subsystem13/1(Out1) -> Mux1/13
  Demux1/11 -> Subsystem11/2(In2)
  Subsystem7/2(Out2) -> Mux/7
  Demux2/5 -> Subsystem5/3(In3)
  Subsystem10/2(Out2) -> Mux/10
  Demux1/1 -> Subsystem1/2(In2)
  Demux2/10 -> Subsystem10/3(In3)
  Demux1/7 -> Subsystem7/2(In2)
  Subsystem16/1(Out1) -> Mux1/16
  Demux/3 -> Subsystem3/1(In1)
  Demux/14 -> Subsystem14/1(In1)
  Subsystem13/2(Out2) -> Mux/13
  Demux/6 -> Subsystem6/1(In1)
  Demux/11 -> Subsystem11/1(In1)
  Mux/1 -> Out1/1
  Subsystem3/2(Out2) -> Mux/3
  Subsystem2/1(Out1) -> Mux1/2
  Subsystem16/2(Out2) -> Mux/16
  Subsystem9/2(Out2) -> Mux/9
  Subsystem10/1(Out1) -> Mux1/10
  Subsystem6/2(Out2) -> Mux/6
  Demux/2 -> Subsystem2/1(In1)
  Demux1/12 -> Subsystem12/2(In2)
  Demux1/15 -> Subsystem15/2(In2)
  Demux2/14 -> Subsystem14/3(In3)
  Demux1/9 -> Subsystem9/2(In2)
  Subsystem4/1(Out1) -> Mux1/4
  Demux1/8 -> Subsystem8/2(In2)
  Demux/12 -> Subsystem12/1(In1)
  Subsystem3/1(Out1) -> Mux1/3
  In1/1 -> Demux2/1
  In2/1 -> Demux1/1
  Demux/8 -> Subsystem8/1(In1)
  Demux2/16 -> Subsystem16/3(In3)
  Demux1/6 -> Subsystem6/2(In2)
  Subsystem14/2(Out2) -> Mux/14
  Demux1/4 -> Subsystem4/2(In2)
  Demux/16 -> Subsystem16/1(In1)
  Subsystem9/1(Out1) -> Mux1/9
  Demux/4 -> Subsystem4/1(In1)
  Demux/15 -> Subsystem15/1(In1)
  Subsystem5/2(Out2) -> Mux/5
  Demux/1 -> Subsystem1/1(In1)
  Demux1/5 -> Subsystem5/2(In2)
  Subsystem15/1(Out1) -> Mux1/15
  Demux/10 -> Subsystem10/1(In1)
  Subsystem15/2(Out2) -> Mux/15
  Demux2/9 -> Subsystem9/3(In3)
  Subsystem6/1(Out1) -> Mux1/6
  Subsystem8/2(Out2) -> Mux/8
  Subsystem8/1(Out1) -> Mux1/8
  Demux2/7 -> Subsystem7/3(In3)
  In3/1 -> Demux/1
  Subsystem11/1(Out1) -> Mux1/11
  Demux1/3 -> Subsystem3/2(In2)
  Demux2/4 -> Subsystem4/3(In3)
  Demux/5 -> Subsystem5/1(In1)

== system wtm2/Subsystem20 ==
  In2 : Inport
  In1 : Inport  Port=2
  In3 : Inport  Port=3
  Demux : Demux  Outputs=16
  Demux1 : Demux  Outputs=16
  Mux : Mux  Inputs=16
  Subsystem4 : Subsystem
  Subsystem5 : Subsystem
  Subsystem6 : Subsystem
  Subsystem7 : Subsystem
  Out1 : Outport
  Out2 : Outport  Port=2
  wires:
  Demux/11 -> Subsystem5/3(In3)
  Subsystem4/4(Out4) -> Mux/15
  Demux1/4 -> Subsystem7/9(In9)
  Demux/14 -> Subsystem4/2(In2)
  Subsystem7/4(Out4) -> Mux/3
  Subsystem7/1(Out1) -> Out1/1
  Subsystem7/3(Out3) -> Mux/2
  Demux/3 -> Subsystem7/3(In3)
  Demux/15 -> Subsystem4/3(In3)
  Subsystem6/1(Out1) -> Subsystem7/5(In5)
  In3/1 -> Demux1/1
  Subsystem4/5(Out5) -> Mux/16
  Subsystem4/3(Out3) -> Mux/14
  Demux1/15 -> Subsystem4/8(In8)
  Subsystem5/4(Out4) -> Mux/11
  Subsystem5/1(Out1) -> Subsystem6/5(In5)
  Subsystem5/3(Out3) -> Mux/10
  Demux1/16 -> Subsystem4/9(In9)
  Demux/9 -> Subsystem5/1(In1)
  Subsystem7/5(Out5) -> Mux/4
  Demux1/3 -> Subsystem7/8(In8)
  Demux1/9 -> Subsystem5/6(In6)
  Subsystem6/5(Out5) -> Mux/8
  Demux/1 -> Subsystem7/1(In1)
  Demux1/13 -> Subsystem4/6(In6)
  Demux/5 -> Subsystem6/1(In1)
  Demux1/7 -> Subsystem6/8(In8)
  In2/1 -> Demux/1
  Demux1/12 -> Subsystem5/9(In9)
  Subsystem6/4(Out4) -> Mux/7
  Subsystem5/5(Out5) -> Mux/12
  Mux/1 -> Out2/1
  Subsystem6/3(Out3) -> Mux/6
  Demux1/8 -> Subsystem6/9(In9)
  Demux/12 -> Subsystem5/4(In4)
  Subsystem4/1(Out1) -> Subsystem5/5(In5)
  Demux/6 -> Subsystem6/2(In2)
  Subsystem6/2(Out2) -> Mux/5
  Demux1/1 -> Subsystem7/6(In6)
  Demux/8 -> Subsystem6/4(In4)
  Demux1/5 -> Subsystem6/6(In6)
  Demux/7 -> Subsystem6/3(In3)
  Demux/4 -> Subsystem7/4(In4)
  Demux/10 -> Subsystem5/2(In2)
  Subsystem5/2(Out2) -> Mux/9
  Demux/2 -> Subsystem7/2(In2)
  Demux1/6 -> Subsystem6/7(In7)
  Subsystem7/2(Out2) -> Mux/1
  Subsystem4/2(Out2) -> Mux/13
  Demux/13 -> Subsystem4/1(In1)
  Demux1/11 -> Subsystem5/8(In8)
  Demux1/2 -> Subsystem7/7(In7)
  Demux1/14 -> Subsystem4/7(In7)
  Demux/16 -> Subsystem4/4(In4)
  Demux1/10 -> Subsystem5/7(In7)
  In1/1 -> Subsystem4/5(In5)

== system wtm2/Subsystem21 ==
  In2 : Inport
  In1 : Inport  Port=2
  In3 : Inport  Port=3
  Demux : Demux  Outputs=16
  Demux1 : Demux  Outputs=16
  Mux : Mux  Inputs=16
  Subsystem4 : Subsystem
  Subsystem5 : Subsystem
  Subsystem6 : Subsystem
  Subsystem7 : Subsystem
  Out1 : Outport
  Out2 : Outport  Port=2
  wires:
  Demux/11 -> Subsystem5/3(In3)
  Subsystem4/4(Out4) -> Mux/15
  Demux1/4 -> Subsystem7/9(In9)
  Demux/14 -> Subsystem4/2(In2)
  Subsystem7/4(Out4) -> Mux/3
  Subsystem7/1(Out1) -> Out1/1
  Subsystem7/3(Out3) -> Mux/2
  Demux/3 -> Subsystem7/3(In3)
  Demux/15 -> Subsystem4/3(In3)
  Subsystem6/1(Out1) -> Subsystem7/5(In5)
  In3/1 -> Demux1/1
  Subsystem4/5(Out5) -> Mux/16
  Subsystem4/3(Out3) -> Mux/14
  Demux1/15 -> Subsystem4/8(In8)
  Subsystem5/4(Out4) -> Mux/11
  Subsystem5/1(Out1) -> Subsystem6/5(In5)
  Subsystem5/3(Out3) -> Mux/10
  Demux1/16 -> Subsystem4/9(In9)
  Demux/9 -> Subsystem5/1(In1)
  Subsystem7/5(Out5) -> Mux/4
  Demux1/3 -> Subsystem7/8(In8)
  Demux1/9 -> Subsystem5/6(In6)
  Subsystem6/5(Out5) -> Mux/8
  Demux/1 -> Subsystem7/1(In1)
  Demux1/13 -> Subsystem4/6(In6)
  Demux/5 -> Subsystem6/1(In1)
  Demux1/7 -> Subsystem6/8(In8)
  In2/1 -> Demux/1
  Demux1/12 -> Subsystem5/9(In9)
  Subsystem6/4(Out4) -> Mux/7
  Subsystem5/5(Out5) -> Mux/12
  Mux/1 -> Out2/1
  Subsystem6/3(Out3) -> Mux/6
  Demux1/8 -> Subsystem6/9(In9)
  Demux/12 -> Subsystem5/4(In4)
  Subsystem4/1(Out1) -> Subsystem5/5(In5)
  Demux/6 -> Subsystem6/2(In2)
  Subsystem6/2(Out2) -> Mux/5
  Demux1/1 -> Subsystem7/6(In6)
  Demux/8 -> Subsystem6/4(In4)
  Demux1/5 -> Subsystem6/6(In6)
  Demux/7 -> Subsystem6/3(In3)
  Demux/4 -> Subsystem7/4(In4)
  Demux/10 -> Subsystem5/2(In2)
  Subsystem5/2(Out2) -> Mux/9
  Demux/2 -> Subsystem7/2(In2)
  Demux1/6 -> Subsystem6/7(In7)
  Subsystem7/2(Out2) -> Mux/1
  Subsystem4/2(Out2) -> Mux/13
  Demux/13 -> Subsystem4/1(In1)
  Demux1/11 -> Subsystem5/8(In8)
  Demux1/2 -> Subsystem7/7(In7)
  Demux1/14 -> Subsystem4/7(In7)
  Demux/16 -> Subsystem4/4(In4)
  Demux1/10 -> Subsystem5/7(In7)
  In1/1 -> Subsystem4/5(In5)

== system wtm2/Subsystem3 ==
  In1 : Inport
  In2 : Inport  Port=2
  In3 : Inport  Port=3
  Demux : Demux  Outputs=16
  Demux1 : Demux  Outputs=16
  Demux2 : Demux  Outputs=16
  Mux : Mux  Inputs=16
  Mux1 : Mux  Inputs=16
  Subsystem1 : Subsystem
  Subsystem10 : Subsystem
  Subsystem11 : Subsystem
  Subsystem12 : Subsystem
  Subsystem13 : Subsystem
  Subsystem14 : Subsystem
  Subsystem15 : Subsystem
  Subsystem16 : Subsystem
  Subsystem2 : Subsystem
  Subsystem3 : Subsystem
  Subsystem4 : Subsystem
  Subsystem5 : Subsystem
  Subsystem6 : Subsystem
  Subsystem7 : Subsystem
  Subsystem8 : Subsystem
  Subsystem9 : Subsystem
  Out1 : Outport
  Out2 : Outport  Port=2
  wires:
  Demux2/2 -> Subsystem2/3(In3)
  Demux/9 -> Subsystem9/1(In1)
  Subsystem7/1(Out1) -> Mux1/7
  Subsystem11/2(Out2) -> Mux/11
  Demux2/8 -> Subsystem8/3(In3)
  Subsystem2/2(Out2) -> Mux/2
  Subsystem1/2(Out2) -> Mux/1
  Demux/7 -> Subsystem7/1(In1)
  Demux2/11 -> Subsystem11/3(In3)
  Demux2/1 -> Subsystem1/3(In3)
  Demux1/10 -> Subsystem10/2(In2)
  Demux2/13 -> Subsystem13/3(In3)
  Subsystem4/2(Out2) -> Mux/4
  Demux1/16 -> Subsystem16/2(In2)
  Demux2/15 -> Subsystem15/3(In3)
  Demux2/3 -> Subsystem3/3(In3)
  Demux2/6 -> Subsystem6/3(In3)
  Mux1/1 -> Out2/1
  Demux/13 -> Subsystem13/1(In1)
  Subsystem14/1(Out1) -> Mux1/14
  Demux1/13 -> Subsystem13/2(In2)
  Subsystem12/1(Out1) -> Mux1/12
  Subsystem1/1(Out1) -> Mux1/1
  Demux1/2 -> Subsystem2/2(In2)
  Subsystem12/2(Out2) -> Mux/12
  Subsystem5/1(Out1) -> Mux1/5
  Demux2/12 -> Subsystem12/3(In3)
  Demux1/14 -> Subsystem14/2(In2)
  Subsystem13/1(Out1) -> Mux1/13
  Demux1/11 -> Subsystem11/2(In2)
  Subsystem7/2(Out2) -> Mux/7
  Demux2/5 -> Subsystem5/3(In3)
  Subsystem10/2(Out2) -> Mux/10
  Demux1/1 -> Subsystem1/2(In2)
  Demux2/10 -> Subsystem10/3(In3)
  Demux1/7 -> Subsystem7/2(In2)
  Subsystem16/1(Out1) -> Mux1/16
  Demux/3 -> Subsystem3/1(In1)
  Demux/14 -> Subsystem14/1(In1)
  Subsystem13/2(Out2) -> Mux/13
  Demux/6 -> Subsystem6/1(In1)
  Demux/11 -> Subsystem11/1(In1)
  Mux/1 -> Out1/1
  Subsystem3/2(Out2) -> Mux/3
  Subsystem2/1(Out1) -> Mux1/2
  Subsystem16/2(Out2) -> Mux/16
  Subsystem9/2(Out2) -> Mux/9
  Subsystem10/1(Out1) -> Mux1/10
  Subsystem6/2(Out2) -> Mux/6
  Demux/2 -> Subsystem2/1(In1)
  Demux1/12 -> Subsystem12/2(In2)
  Demux1/15 -> Subsystem15/2(In2)
  Demux2/14 -> Subsystem14/3(In3)
  Demux1/9 -> Subsystem9/2(In2)
  Subsystem4/1(Out1) -> Mux1/4
  Demux1/8 -> Subsystem8/2(In2)
  Demux/12 -> Subsystem12/1(In1)
  Subsystem3/1(Out1) -> Mux1/3
  In1/1 -> Demux2/1
  In2/1 -> Demux1/1
  Demux/8 -> Subsystem8/1(In1)
  Demux2/16 -> Subsystem16/3(In3)
  Demux1/6 -> Subsystem6/2(In2)
  Subsystem14/2(Out2) -> Mux/14
  Demux1/4 -> Subsystem4/2(In2)
  Demux/16 -> Subsystem16/1(In1)
  Subsystem9/1(Out1) -> Mux1/9
  Demux/4 -> Subsystem4/1(In1)
  Demux/15 -> Subsystem15/1(In1)
  Subsystem5/2(Out2) -> Mux/5
  Demux/1 -> Subsystem1/1(In1)
  Demux1/5 -> Subsystem5/2(In2)
  Subsystem15/1(Out1) -> Mux1/15
  Demux/10 -> Subsystem10/1(In1)
  Subsystem15/2(Out2) -> Mux/15
  Demux2/9 -> Subsystem9/3(In3)
  Subsystem6/1(Out1) -> Mux1/6
  Subsystem8/2(Out2) -> Mux/8
  Subsystem8/1(Out1) -> Mux1/8
  Demux2/7 -> Subsystem7/3(In3)
  In3/1 -> Demux/1
  Subsystem11/1(Out1) -> Mux1/11
  Demux1/3 -> Subsystem3/2(In2)
  Demux2/4 -> Subsystem4/3(In3)
  Demux/5 -> Subsystem5/1(In1)

== system wtm2/Subsystem4 ==
  In1 : Inport
  In2 : Inport  Port=2
  In3 : Inport  Port=3
  Demux : Demux  Outputs=16
  Demux1 : Demux  Outputs=16
  Demux2 : Demux  Outputs=16
  Mux : Mux  Inputs=16
  Mux1 : Mux  Inputs=16
  Subsystem1 : Subsystem
  Subsystem10 : Subsystem
  Subsystem11 : Subsystem
  Subsystem12 : Subsystem
  Subsystem13 : Subsystem
  Subsystem14 : Subsystem
  Subsystem15 : Subsystem
  Subsystem16 : Subsystem
  Subsystem2 : Subsystem
  Subsystem3 : Subsystem
  Subsystem4 : Subsystem
  Subsystem5 : Subsystem
  Subsystem6 : Subsystem
  Subsystem7 : Subsystem
  Subsystem8 : Subsystem
  Subsystem9 : Subsystem
  Out1 : Outport
  Out2 : Outport  Port=2
  wires:
  Demux2/2 -> Subsystem2/3(In3)
  Demux/9 -> Subsystem9/1(In1)
  Subsystem7/1(Out1) -> Mux1/7
  Subsystem11/2(Out2) -> Mux/11
  Demux2/8 -> Subsystem8/3(In3)
  Subsystem2/2(Out2) -> Mux/2
  Subsystem1/2(Out2) -> Mux/1
  Demux/7 -> Subsystem7/1(In1)
  Demux2/11 -> Subsystem11/3(In3)
  Demux2/1 -> Subsystem1/3(In3)
  Demux1/10 -> Subsystem10/2(In2)
  Demux2/13 -> Subsystem13/3(In3)
  Subsystem4/2(Out2) -> Mux/4
  Demux1/16 -> Subsystem16/2(In2)
  Demux2/15 -> Subsystem15/3(In3)
  Demux2/3 -> Subsystem3/3(In3)
  Demux2/6 -> Subsystem6/3(In3)
  Mux1/1 -> Out2/1
  Demux/13 -> Subsystem13/1(In1)
  Subsystem14/1(Out1) -> Mux1/14
  Demux1/13 -> Subsystem13/2(In2)
  Subsystem12/1(Out1) -> Mux1/12
  Subsystem1/1(Out1) -> Mux1/1
  Demux1/2 -> Subsystem2/2(In2)
  Subsystem12/2(Out2) -> Mux/12
  Subsystem5/1(Out1) -> Mux1/5
  Demux2/12 -> Subsystem12/3(In3)
  Demux1/14 -> Subsystem14/2(In2)
  Subsystem13/1(Out1) -> Mux1/13
  Demux1/11 -> Subsystem11/2(In2)
  Subsystem7/2(Out2) -> Mux/7
  Demux2/5 -> Subsystem5/3(In3)
  Subsystem10/2(Out2) -> Mux/10
  Demux1/1 -> Subsystem1/2(In2)
  Demux2/10 -> Subsystem10/3(In3)
  Demux1/7 -> Subsystem7/2(In2)
  Subsystem16/1(Out1) -> Mux1/16
  Demux/3 -> Subsystem3/1(In1)
  Demux/14 -> Subsystem14/1(In1)
  Subsystem13/2(Out2) -> Mux/13
  Demux/6 -> Subsystem6/1(In1)
  Demux/11 -> Subsystem11/1(In1)
  Mux/1 -> Out1/1
  Subsystem3/2(Out2) -> Mux/3
  Subsystem2/1(Out1) -> Mux1/2
  Subsystem16/2(Out2) -> Mux/16
  Subsystem9/2(Out2) -> Mux/9
  Subsystem10/1(Out1) -> Mux1/10
  Subsystem6/2(Out2) -> Mux/6
  Demux/2 -> Subsystem2/1(In1)
  Demux1/12 -> Subsystem12/2(In2)
  Demux1/15 -> Subsystem15/2(In2)
  Demux2/14 -> Subsystem14/3(In3)
  Demux1/9 -> Subsystem9/2(In2)
  Subsystem4/1(Out1) -> Mux1/4
  Demux1/8 -> Subsystem8/2(In2)
  Demux/12 -> Subsystem12/1(In1)
  Subsystem3/1(Out1) -> Mux1/3
  In1/1 -> Demux2/1
  In2/1 -> Demux1/1
  Demux/8 -> Subsystem8/1(In1)
  Demux2/16 -> Subsystem16/3(In3)
  Demux1/6 -> Subsystem6/2(In2)
  Subsystem14/2(Out2) -> Mux/14
  Demux1/4 -> Subsystem4/2(In2)
  Demux/16 -> Subsystem16/1(In1)
  Subsystem9/1(Out1) -> Mux1/9
  Demux/4 -> Subsystem4/1(In1)
  Demux/15 -> Subsystem15/1(In1)
  Subsystem5/2(Out2) -> Mux/5
  Demux/1 -> Subsystem1/1(In1)
  Demux1/5 -> Subsystem5/2(In2)
  Subsystem15/1(Out1) -> Mux1/15
  Demux/10 -> Subsystem10/1(In1)
  Subsystem15/2(Out2) -> Mux/15
  Demux2/9 -> Subsystem9/3(In3)
  Subsystem6/1(Out1) -> Mux1/6
  Subsystem8/2(Out2) -> Mux/8
  Subsystem8/1(Out1) -> Mux1/8
  Demux2/7 -> Subsystem7/3(In3)
  In3/1 -> Demux/1
  Subsystem11/1(Out1) -> Mux1/11
  Demux1/3 -> Subsystem3/2(In2)
  Demux2/4 -> Subsystem4/3(In3)
  Demux/5 -> Subsystem5/1(In1)

== system wtm2/Subsystem5 ==
  In1 : Inport
  In2 : Inport  Port=2
  In3 : Inport  Port=3
  Demux : Demux  Outputs=16
  Demux1 : Demux  Outputs=16
  Demux2 : Demux  Outputs=16
  Mux : Mux  Inputs=16
  Mux1 : Mux  Inputs=16
  Subsystem1 : Subsystem
  Subsystem10 : Subsystem
  Subsystem11 : Subsystem
  Subsystem12 : Subsystem
  Subsystem13 : Subsystem
  Subsystem14 : Subsystem
  Subsystem15 : Subsystem
  Subsystem16 : Subsystem
  Subsystem2 : Subsystem
  Subsystem3 : Subsystem
  Subsystem4 : Subsystem
  Subsystem5 : Subsystem
  Subsystem6 : Subsystem
  Subsystem7 : Subsystem
  Subsystem8 : Subsystem
  Subsystem9 : Subsystem
  Out1 : Outport
  Out2 : Outport  Port=2
  wires:
  Demux2/2 -> Subsystem2/3(In3)
  Demux/9 -> Subsystem9/1(In1)
  Subsystem7/1(Out1) -> Mux1/7
  Subsystem11/2(Out2) -> Mux/11
  Demux2/8 -> Subsystem8/3(In3)
  Subsystem2/2(Out2) -> Mux/2
  Subsystem1/2(Out2) -> Mux/1
  Demux/7 -> Subsystem7/1(In1)
  Demux2/11 -> Subsystem11/3(In3)
  Demux2/1 -> Subsystem1/3(In3)
  Demux1/10 -> Subsystem10/2(In2)
  Demux2/13 -> Subsystem13/3(In3)
  Subsystem4/2(Out2) -> Mux/4
  Demux1/16 -> Subsystem16/2(In2)
  Demux2/15 -> Subsystem15/3(In3)
  Demux2/3 -> Subsystem3/3(In3)
  Demux2/6 -> Subsystem6/3(In3)
  Mux1/1 -> Out2/1
  Demux/13 -> Subsystem13/1(In1)
  Subsystem14/1(Out1) -> Mux1/14
  Demux1/13 -> Subsystem13/2(In2)
  Subsystem12/1(Out1) -> Mux1/12
  Subsystem1/1(Out1) -> Mux1/1
  Demux1/2 -> Subsystem2/2(In2)
  Subsystem12/2(Out2) -> Mux/12
  Subsystem5/1(Out1) -> Mux1/5
  Demux2/12 -> Subsystem12/3(In3)
  Demux1/14 -> Subsystem14/2(In2)
  Subsystem13/1(Out1) -> Mux1/13
  Demux1/11 -> Subsystem11/2(In2)
  Subsystem7/2(Out2) -> Mux/7
  Demux2/5 -> Subsystem5/3(In3)
  Subsystem10/2(Out2) -> Mux/10
  Demux1/1 -> Subsystem1/2(In2)
  Demux2/10 -> Subsystem10/3(In3)
  Demux1/7 -> Subsystem7/2(In2)
  Subsystem16/1(Out1) -> Mux1/16
  Demux/3 -> Subsystem3/1(In1)
  Demux/14 -> Subsystem14/1(In1)
  Subsystem13/2(Out2) -> Mux/13
  Demux/6 -> Subsystem6/1(In1)
  Demux/11 -> Subsystem11/1(In1)
  Mux/1 -> Out1/1
  Subsystem3/2(Out2) -> Mux/3
  Subsystem2/1(Out1) -> Mux1/2
  Subsystem16/2(Out2) -> Mux/16
  Subsystem9/2(Out2) -> Mux/9
  Subsystem10/1(Out1) -> Mux1/10
  Subsystem6/2(Out2) -> Mux/6
  Demux/2 -> Subsystem2/1(In1)
  Demux1/12 -> Subsystem12/2(In2)
  Demux1/15 -> Subsystem15/2(In2)
  Demux2/14 -> Subsystem14/3(In3)
  Demux1/9 -> Subsystem9/2(In2)
  Subsystem4/1(Out1) -> Mux1/4
  Demux1/8 -> Subsystem8/2(In2)
  Demux/12 -> Subsystem12/1(In1)
  Subsystem3/1(Out1) -> Mux1/3
  In1/1 -> Demux2/1
  In2/1 -> Demux1/1
  Demux/8 -> Subsystem8/1(In1)
  Demux2/16 -> Subsystem16/3(In3)
  Demux1/6 -> Subsystem6/2(In2)
  Subsystem14/2(Out2) -> Mux/14
  Demux1/4 -> Subsystem4/2(In2)
  Demux/16 -> Subsystem16/1(In1)
  Subsystem9/1(Out1) -> Mux1/9
  Demux/4 -> Subsystem4/1(In1)
  Demux/15 -> Subsystem15/1(In1)
  Subsystem5/2(Out2) -> Mux/5
  Demux/1 -> Subsystem1/1(In1)
  Demux1/5 -> Subsystem5/2(In2)
  Subsystem15/1(Out1) -> Mux1/15
  Demux/10 -> Subsystem10/1(In1)
  Subsystem15/2(Out2) -> Mux/15
  Demux2/9 -> Subsystem9/3(In3)
  Subsystem6/1(Out1) -> Mux1/6
  Subsystem8/2(Out2) -> Mux/8
  Subsystem8/1(Out1) -> Mux1/8
  Demux2/7 -> Subsystem7/3(In3)
  In3/1 -> Demux/1
  Subsystem11/1(Out1) -> Mux1/11
  Demux1/3 -> Subsystem3/2(In2)
  Demux2/4 -> Subsystem4/3(In3)
  Demux/5 -> Subsystem5/1(In1)

== system wtm2/Subsystem6 ==
  In1 : Inport
  In2 : Inport  Port=2
  In3 : Inport  Port=3
  Demux : Demux  Outputs=16
  Demux1 : Demux  Outputs=16
  Demux2 : Demux  Outputs=16
  Mux : Mux  Inputs=16
  Mux1 : Mux  Inputs=16
  Subsystem1 : Subsystem
  Subsystem10 : Subsystem
  Subsystem11 : Subsystem
  Subsystem12 : Subsystem
  Subsystem13 : Subsystem
  Subsystem14 : Subsystem
  Subsystem15 : Subsystem
  Subsystem16 : Subsystem
  Subsystem2 : Subsystem
  Subsystem3 : Subsystem
  Subsystem4 : Subsystem
  Subsystem5 : Subsystem
  Subsystem6 : Subsystem
  Subsystem7 : Subsystem
  Subsystem8 : Subsystem
  Subsystem9 : Subsystem
  Out1 : Outport
  Out2 : Outport  Port=2
  wires:
  Demux2/2 -> Subsystem2/3(In3)
  Demux/9 -> Subsystem9/1(In1)
  Subsystem7/1(Out1) -> Mux1/7
  Subsystem11/2(Out2) -> Mux/11
  Demux2/8 -> Subsystem8/3(In3)
  Subsystem2/2(Out2) -> Mux/2
  Subsystem1/2(Out2) -> Mux/1
  Demux/7 -> Subsystem7/1(In1)
  Demux2/11 -> Subsystem11/3(In3)
  Demux2/1 -> Subsystem1/3(In3)
  Demux1/10 -> Subsystem10/2(In2)
  Demux2/13 -> Subsystem13/3(In3)
  Subsystem4/2(Out2) -> Mux/4
  Demux1/16 -> Subsystem16/2(In2)
  Demux2/15 -> Subsystem15/3(In3)
  Demux2/3 -> Subsystem3/3(In3)
  Demux2/6 -> Subsystem6/3(In3)
  Mux1/1 -> Out2/1
  Demux/13 -> Subsystem13/1(In1)
  Subsystem14/1(Out1) -> Mux1/14
  Demux1/13 -> Subsystem13/2(In2)
  Subsystem12/1(Out1) -> Mux1/12
  Subsystem1/1(Out1) -> Mux1/1
  Demux1/2 -> Subsystem2/2(In2)
  Subsystem12/2(Out2) -> Mux/12
  Subsystem5/1(Out1) -> Mux1/5
  Demux2/12 -> Subsystem12/3(In3)
  Demux1/14 -> Subsystem14/2(In2)
  Subsystem13/1(Out1) -> Mux1/13
  Demux1/11 -> Subsystem11/2(In2)
  Subsystem7/2(Out2) -> Mux/7
  Demux2/5 -> Subsystem5/3(In3)
  Subsystem10/2(Out2) -> Mux/10
  Demux1/1 -> Subsystem1/2(In2)
  Demux2/10 -> Subsystem10/3(In3)
  Demux1/7 -> Subsystem7/2(In2)
  Subsystem16/1(Out1) -> Mux1/16
  Demux/3 -> Subsystem3/1(In1)
  Demux/14 -> Subsystem14/1(In1)
  Subsystem13/2(Out2) -> Mux/13
  Demux/6 -> Subsystem6/1(In1)
  Demux/11 -> Subsystem11/1(In1)
  Mux/1 -> Out1/1
  Subsystem3/2(Out2) -> Mux/3
  Subsystem2/1(Out1) -> Mux1/2
  Subsystem16/2(Out2) -> Mux/16
  Subsystem9/2(Out2) -> Mux/9
  Subsystem10/1(Out1) -> Mux1/10
  Subsystem6/2(Out2) -> Mux/6
  Demux/2 -> Subsystem2/1(In1)
  Demux1/12 -> Subsystem12/2(In2)
  Demux1/15 -> Subsystem15/2(In2)
  Demux2/14 -> Subsystem14/3(In3)
  Demux1/9 -> Subsystem9/2(In2)
  Subsystem4/1(Out1) -> Mux1/4
  Demux1/8 -> Subsystem8/2(In2)
  Demux/12 -> Subsystem12/1(In1)
  Subsystem3/1(Out1) -> Mux1/3
  In1/1 -> Demux2/1
  In2/1 -> Demux1/1
  Demux/8 -> Subsystem8/1(In1)
  Demux2/16 -> Subsystem16/3(In3)
  Demux1/6 -> Subsystem6/2(In2)
  Subsystem14/2(Out2) -> Mux/14
  Demux1/4 -> Subsystem4/2(In2)
  Demux/16 -> Subsystem16/1(In1)
  Subsystem9/1(Out1) -> Mux1/9
  Demux/4 -> Subsystem4/1(In1)
  Demux/15 -> Subsystem15/1(In1)
  Subsystem5/2(Out2) -> Mux/5
  Demux/1 -> Subsystem1/1(In1)
  Demux1/5 -> Subsystem5/2(In2)
  Subsystem15/1(Out1) -> Mux1/15
  Demux/10 -> Subsystem10/1(In1)
  Subsystem15/2(Out2) -> Mux/15
  Demux2/9 -> Subsystem9/3(In3)
  Subsystem6/1(Out1) -> Mux1/6
  Subsystem8/2(Out2) -> Mux/8
  Subsystem8/1(Out1) -> Mux1/8
  Demux2/7 -> Subsystem7/3(In3)
  In3/1 -> Demux/1
  Subsystem11/1(Out1) -> Mux1/11
  Demux1/3 -> Subsystem3/2(In2)
  Demux2/4 -> Subsystem4/3(In3)
  Demux/5 -> Subsystem5/1(In1)

== system wtm2/Subsystem7 ==
  In1 : Inport
  Constant : Constant  Value=0  OutDataTypeStr=boolean
  Demux : Demux  Outputs=16
  Display : Display
  Mux : Mux  Inputs=16
  Out2 : Outport
  wires:
  Demux/5 -> Mux/6
  Demux/6 -> Mux/7
  Demux/4 -> Mux/5
  Demux/10 -> Mux/11
  In1/1 -> Demux/1
  Constant/1 -> Mux/1
  Demux/15 -> Mux/16
  Mux/1 -> Out2/1
  Demux/1 -> Mux/2
  Demux/9 -> Mux/10
  Demux/2 -> Mux/3
  Demux/11 -> Mux/12
  Demux/12 -> Mux/13
  Demux/14 -> Mux/15
  Demux/13 -> Mux/14
  Demux/3 -> Mux/4
  Demux/8 -> Mux/9
  Demux/7 -> Mux/8
  Demux/16 -> Display/1
